simulink model "Problem1"  (R2020b)
settings: Solver=VariableStepAuto  StartTime=0.0  StopTime=10.0  RelTol=1e-3
model workspace (MAT data in the model file):
  b = Simulink.Parameter
  b.Value = 50
  b.DataType = 'auto'
  b.Dimensions = [1 1]
  k1 = Simulink.Parameter
  k1.Value = 50
  k1.DataType = 'auto'
  k1.Dimensions = [1 1]
  k12 = Simulink.Parameter
  k12.Value = 500
  k12.DataType = 'auto'
  k12.Dimensions = [1 1]
  m1 = Simulink.Parameter
  m1.Value = 100
  m1.DataType = 'auto'
  m1.Dimensions = [1 1]
  m2 = Simulink.Parameter
  m2.Value = 5
  m2.DataType = 'auto'
  m2.Dimensions = [1 1]
settings Model: Creator=amolg  LastModifiedBy=amolg

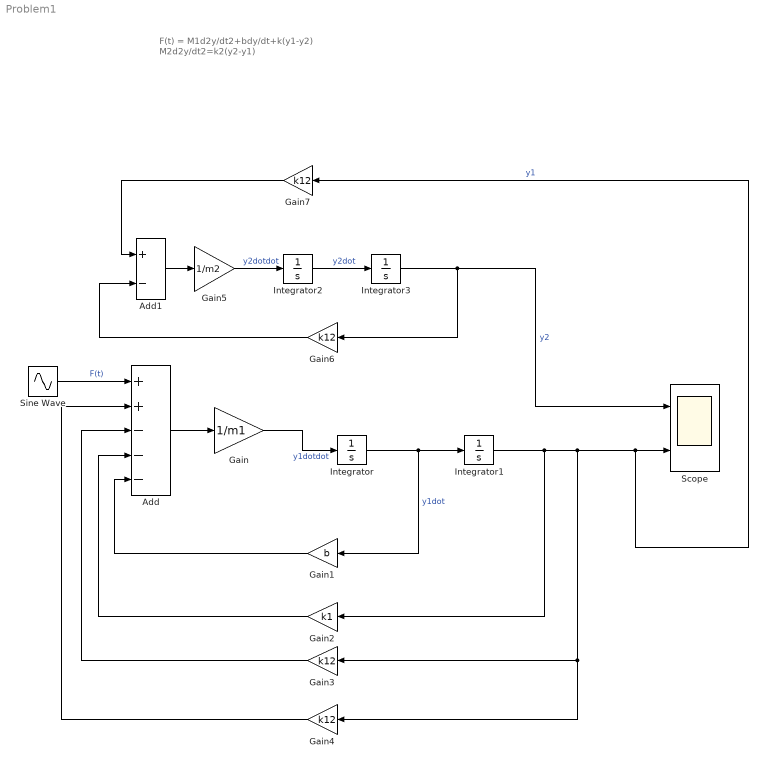
== system Problem1 ==
  note: F(t) = M1d2y/dt2+bdy/dt+k(y1-y2)
      | M2d2y/dt2=k2(y2-y1)
  Add : Sum  Inputs=++---
  Add1 : Sum  Inputs=+-
  Gain : Gain  Gain=1/m1
  Gain1 : Gain  Gain=b
  Gain2 : Gain  Gain=k1
  Gain{3..4,6..7} (4 alike) : Gain  Gain=k12
  Gain5 : Gain  Gain=1/m2
  Integrator{,1..3} (4 alike) : Integrator
  Scope : Scope  NumInputPorts=2
  Sine Wave : Sin  Amplitude=2  Frequency=10  SampleTime=0
  wires:
  Gain/1 -> Integrator/1  "y1dotdot"
  Add/1 -> Gain/1
  Integrator/1 -> Gain1/1, Integrator1/1  "y1dot"
  Integrator1/1 -> Gain2/1, Gain7/1, Scope/2, Gain3/1, Gain4/1  "y1"
  Gain5/1 -> Integrator2/1  "y2dotdot"
  Gain2/1 -> Add/4
  Sine Wave/1 -> Add/1  "F(t)"
  Gain7/1 -> Add1/1
  Gain3/1 -> Add/3
  Add1/1 -> Gain5/1
  Integrator2/1 -> Integrator3/1  "y2dot"
  Integrator3/1 -> Gain6/1, Scope/1  "y2"
  Gain4/1 -> Add/2
  Gain1/1 -> Add/5
  Gain6/1 -> Add1/2
